simulink model "EVX_Car_Model"  (R2018b)
settings: Solver=VariableStepAuto  StartTime=0.0  StopTime=10.0  RelTol=1e-3
settings Model: Creator=Foster  LastModifiedBy=Foster

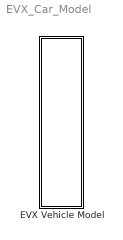
== system EVX_Car_Model ==
  EVX Vehicle Model : Subsystem

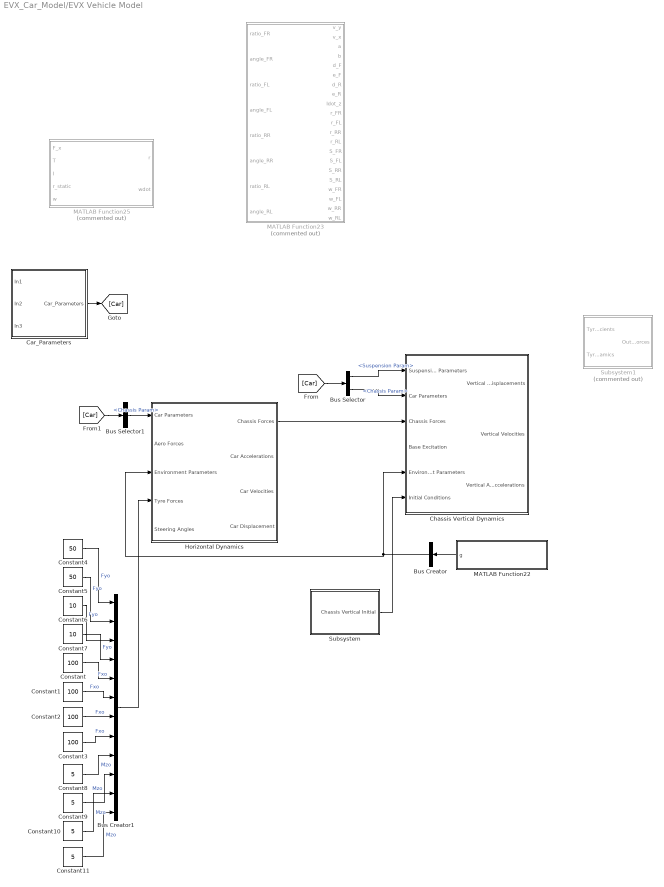
== system EVX_Car_Model/EVX Vehicle Model ==
  Bus Creator : BusCreator  Inputs=1
  Bus Creator1 : BusCreator  Inputs=12
  Bus Selector : BusSelector  OutputSignals=Suspension Param,Chassis Param
  Bus Selector1 : BusSelector  OutputSignals=Chassis Param
  Car_Parameters : Subsystem
  Chassis Vertical Dynamics : Subsystem
  Constant{,1..3} (4 alike) : Constant  Value=100
  Constant{8..11} (4 alike) : Constant  Value=5
  Constant4 : Constant  Value=50
  Constant5 : Constant  Value=50
  Constant6 : Constant  Value=10
  Constant7 : Constant  Value=10
  Horizontal Dynamics : Subsystem
  MATLAB Function22 : MATLAB Function  TreatAsAtomicUnit=on
  MATLAB Function23 : MATLAB Function  Commented=on  TreatAsAtomicUnit=on
  MATLAB Function25 : MATLAB Function  Commented=on  TreatAsAtomicUnit=on
  Subsystem : Subsystem
  Subsystem1 : Subsystem  Commented=on
  wires:
  Subsystem/1(Chassis Vertical Initial) -> Chassis Vertical Dynamics/6(Initial Conditions)
  Constant7/1 -> Bus Creator1/4  "Fyo"
  Constant6/1 -> Bus Creator1/3  "Fyo"
  Constant11/1 -> Bus Creator1/12  "Mzo"
  Bus Creator1/1 -> Horizontal Dynamics/4(Tyre Forces)
  MATLAB Function22/1(g) -> Bus Creator/1
  Constant9/1 -> Bus Creator1/10  "Mzo"
  Constant4/1 -> Bus Creator1/1  "Fyo"
  Bus Selector/1 -> Chassis Vertical Dynamics/1(Suspension Parameters)  "<Suspension Param>"
  Constant3/1 -> Bus Creator1/8  "Fxo"
  Bus Selector1/1 -> Horizontal Dynamics/1(Car Parameters)  "<Chassis Param>"
  [Car] -> Bus Selector/1
  Constant10/1 -> Bus Creator1/11  "Mzo"
  Bus Selector/2 -> Chassis Vertical Dynamics/2(Car Parameters)  "<Chassis Param>"
  Car_Parameters/1(Car_Parameters) -> [Car]
  Horizontal Dynamics/1(Chassis Forces) -> Chassis Vertical Dynamics/3(Chassis Forces)
  [Car] -> Bus Selector1/1
  Constant1/1 -> Bus Creator1/6  "Fxo"
  Constant2/1 -> Bus Creator1/7  "Fxo"
  Bus Creator/1 -> Chassis Vertical Dynamics/5(Environment Parameters), Horizontal Dynamics/3(Environment Parameters)
  Constant/1 -> Bus Creator1/5  "Fxo"
  Constant5/1 -> Bus Creator1/2  "Fyo"
  Constant8/1 -> Bus Creator1/9  "Mzo"

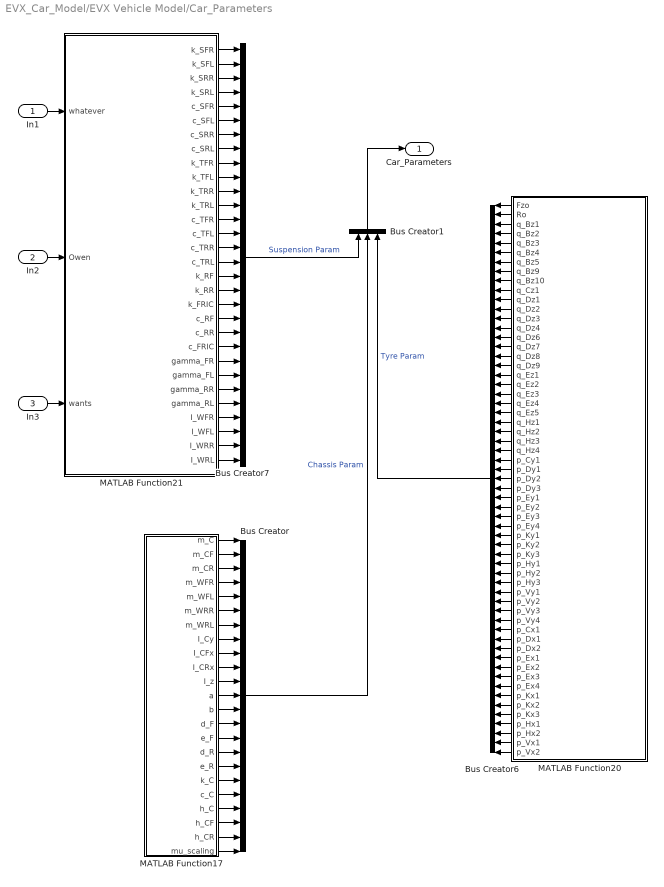
== system EVX_Car_Model/EVX Vehicle Model/Car_Parameters ==
  In1 : Inport
  In2 : Inport  Port=2
  In3 : Inport  Port=3
  Bus Creator : BusCreator  Inputs=23
  Bus Creator1 : BusCreator  Inputs=3
  Bus Creator6 : BusCreator  Inputs=59
  Bus Creator7 : BusCreator  Inputs=30
  MATLAB Function17 : MATLAB Function  TreatAsAtomicUnit=on
  MATLAB Function20 : MATLAB Function  TreatAsAtomicUnit=on
  MATLAB Function21 : MATLAB Function  TreatAsAtomicUnit=on
  Car_Parameters : Outport
  wires:
  In1/1 -> MATLAB Function21/1(whatever)
  In2/1 -> MATLAB Function21/2(Owen)
  In3/1 -> MATLAB Function21/3(wants)
  MATLAB Function21/1(k_SFR) -> Bus Creator7/1
  MATLAB Function21/2(k_SFL) -> Bus Creator7/2
  MATLAB Function21/3(k_SRR) -> Bus Creator7/3
  MATLAB Function21/4(k_SRL) -> Bus Creator7/4
  MATLAB Function21/5(c_SFR) -> Bus Creator7/5
  MATLAB Function21/6(c_SFL) -> Bus Creator7/6
  MATLAB Function21/7(c_SRR) -> Bus Creator7/7
  MATLAB Function21/8(c_SRL) -> Bus Creator7/8
  MATLAB Function21/9(k_TFR) -> Bus Creator7/9
  MATLAB Function21/10(k_TFL) -> Bus Creator7/10
  MATLAB Function21/11(k_TRR) -> Bus Creator7/11
  MATLAB Function21/12(k_TRL) -> Bus Creator7/12
  MATLAB Function21/13(c_TFR) -> Bus Creator7/13
  MATLAB Function21/14(c_TFL) -> Bus Creator7/14
  MATLAB Function21/15(c_TRR) -> Bus Creator7/15
  MATLAB Function21/16(c_TRL) -> Bus Creator7/16
  MATLAB Function21/17(k_RF) -> Bus Creator7/17
  MATLAB Function21/18(k_RR) -> Bus Creator7/18
  MATLAB Function21/19(k_FRIC) -> Bus Creator7/19
  MATLAB Function21/20(c_RF) -> Bus Creator7/20
  MATLAB Function21/21(c_RR) -> Bus Creator7/21
  MATLAB Function21/22(c_FRIC) -> Bus Creator7/22
  MATLAB Function21/23(gamma_FR) -> Bus Creator7/23
  MATLAB Function21/24(gamma_FL) -> Bus Creator7/24
  MATLAB Function21/25(gamma_RR) -> Bus Creator7/25
  MATLAB Function21/26(gamma_RL) -> Bus Creator7/26
  MATLAB Function21/27(I_WFR) -> Bus Creator7/27
  MATLAB Function21/28(I_WFL) -> Bus Creator7/28
  MATLAB Function21/29(I_WRR) -> Bus Creator7/29
  MATLAB Function21/30(I_WRL) -> Bus Creator7/30
  MATLAB Function17/1(m_C) -> Bus Creator/1
  MATLAB Function17/2(m_CF) -> Bus Creator/2
  MATLAB Function17/3(m_CR) -> Bus Creator/3
  MATLAB Function17/4(m_WFR) -> Bus Creator/4
  MATLAB Function17/5(m_WFL) -> Bus Creator/5
  MATLAB Function17/6(m_WRR) -> Bus Creator/6
  MATLAB Function17/7(m_WRL) -> Bus Creator/7
  MATLAB Function17/8(I_Cy) -> Bus Creator/8
  MATLAB Function17/9(I_CFx) -> Bus Creator/9
  MATLAB Function17/10(I_CRx) -> Bus Creator/10
  MATLAB Function17/11(I_z) -> Bus Creator/11
  MATLAB Function17/12(a) -> Bus Creator/12
  MATLAB Function17/13(b) -> Bus Creator/13
  MATLAB Function17/14(d_F) -> Bus Creator/14
  MATLAB Function17/15(e_F) -> Bus Creator/15
  MATLAB Function17/16(d_R) -> Bus Creator/16
  MATLAB Function17/17(e_R) -> Bus Creator/17
  MATLAB Function17/18(k_C) -> Bus Creator/18
  MATLAB Function17/19(c_C) -> Bus Creator/19
  MATLAB Function17/20(h_C) -> Bus Creator/20
  MATLAB Function17/21(h_CF) -> Bus Creator/21
  MATLAB Function17/22(h_CR) -> Bus Creator/22
  MATLAB Function17/23(mu_scaling) -> Bus Creator/23
  MATLAB Function20/1(Fzo) -> Bus Creator6/1
  MATLAB Function20/59(p_Vx2) -> Bus Creator6/59
  MATLAB Function20/58(p_Vx1) -> Bus Creator6/58
  MATLAB Function20/57(p_Hx2) -> Bus Creator6/57
  MATLAB Function20/56(p_Hx1) -> Bus Creator6/56
  MATLAB Function20/55(p_Kx3) -> Bus Creator6/55
  MATLAB Function20/54(p_Kx2) -> Bus Creator6/54
  MATLAB Function20/53(p_Kx1) -> Bus Creator6/53
  MATLAB Function20/52(p_Ex4) -> Bus Creator6/52
  MATLAB Function20/51(p_Ex3) -> Bus Creator6/51
  MATLAB Function20/50(p_Ex2) -> Bus Creator6/50
  MATLAB Function20/49(p_Ex1) -> Bus Creator6/49
  MATLAB Function20/48(p_Dx2) -> Bus Creator6/48
  MATLAB Function20/47(p_Dx1) -> Bus Creator6/47
  MATLAB Function20/46(p_Cx1) -> Bus Creator6/46
  MATLAB Function20/45(p_Vy4) -> Bus Creator6/45
  MATLAB Function20/44(p_Vy3) -> Bus Creator6/44
  MATLAB Function20/43(p_Vy2) -> Bus Creator6/43
  MATLAB Function20/42(p_Vy1) -> Bus Creator6/42
  MATLAB Function20/41(p_Hy3) -> Bus Creator6/41
  MATLAB Function20/39(p_Hy1) -> Bus Creator6/39
  MATLAB Function20/40(p_Hy2) -> Bus Creator6/40
  MATLAB Function20/38(p_Ky3) -> Bus Creator6/38
  MATLAB Function20/37(p_Ky2) -> Bus Creator6/37
  MATLAB Function20/36(p_Ky1) -> Bus Creator6/36
  MATLAB Function20/35(p_Ey4) -> Bus Creator6/35
  MATLAB Function20/34(p_Ey3) -> Bus Creator6/34
  MATLAB Function20/33(p_Ey2) -> Bus Creator6/33
  MATLAB Function20/32(p_Ey1) -> Bus Creator6/32
  MATLAB Function20/31(p_Dy3) -> Bus Creator6/31
  MATLAB Function20/2(Ro) -> Bus Creator6/2
  MATLAB Function20/3(q_Bz1) -> Bus Creator6/3
  MATLAB Function20/4(q_Bz2) -> Bus Creator6/4
  MATLAB Function20/5(q_Bz3) -> Bus Creator6/5
  MATLAB Function20/6(q_Bz4) -> Bus Creator6/6
  MATLAB Function20/7(q_Bz5) -> Bus Creator6/7
  MATLAB Function20/8(q_Bz9) -> Bus Creator6/8
  MATLAB Function20/9(q_Bz10) -> Bus Creator6/9
  MATLAB Function20/10(q_Cz1) -> Bus Creator6/10
  MATLAB Function20/11(q_Dz1) -> Bus Creator6/11
  MATLAB Function20/12(q_Dz2) -> Bus Creator6/12
  MATLAB Function20/13(q_Dz3) -> Bus Creator6/13
  MATLAB Function20/14(q_Dz4) -> Bus Creator6/14
  MATLAB Function20/15(q_Dz6) -> Bus Creator6/15
  MATLAB Function20/16(q_Dz7) -> Bus Creator6/16
  MATLAB Function20/17(q_Dz8) -> Bus Creator6/17
  MATLAB Function20/18(q_Dz9) -> Bus Creator6/18
  MATLAB Function20/19(q_Ez1) -> Bus Creator6/19
  MATLAB Function20/20(q_Ez2) -> Bus Creator6/20
  MATLAB Function20/21(q_Ez3) -> Bus Creator6/21
  MATLAB Function20/22(q_Ez4) -> Bus Creator6/22
  MATLAB Function20/23(q_Ez5) -> Bus Creator6/23
  MATLAB Function20/24(q_Hz1) -> Bus Creator6/24
  MATLAB Function20/25(q_Hz2) -> Bus Creator6/25
  MATLAB Function20/26(q_Hz3) -> Bus Creator6/26
  MATLAB Function20/27(q_Hz4) -> Bus Creator6/27
  MATLAB Function20/28(p_Cy1) -> Bus Creator6/28
  MATLAB Function20/29(p_Dy1) -> Bus Creator6/29
  MATLAB Function20/30(p_Dy2) -> Bus Creator6/30
  Bus Creator7/1 -> Bus Creator1/1  "Suspension Param"
  Bus Creator/1 -> Bus Creator1/2  "Chassis Param"
  Bus Creator6/1 -> Bus Creator1/3  "Tyre Param"
  Bus Creator1/1 -> Car_Parameters/1

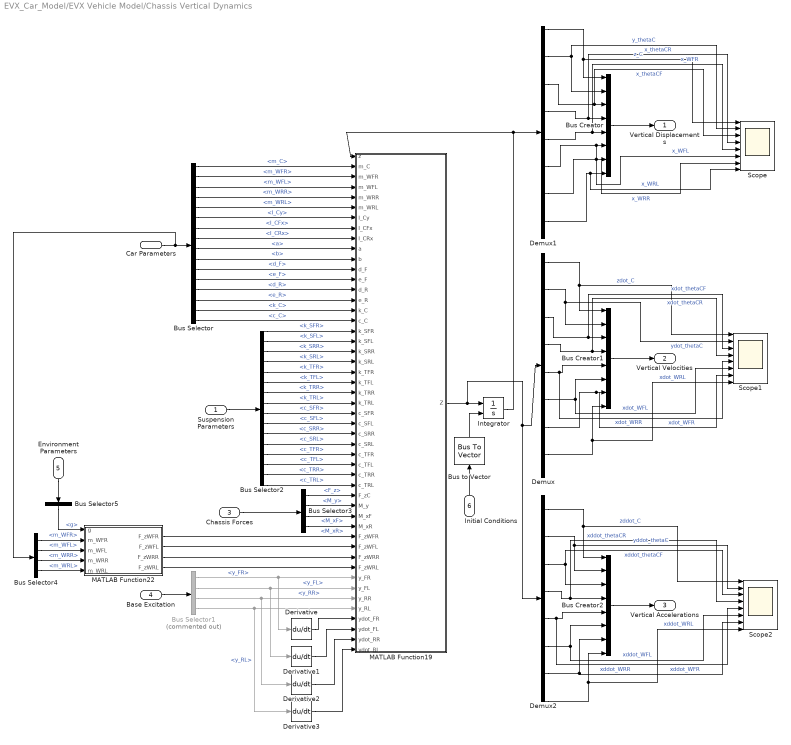
== system EVX_Car_Model/EVX Vehicle Model/Chassis Vertical Dynamics ==
  Suspension Parameters : Inport
  Car Parameters : Inport  Port=2
  Chassis Forces : Inport  Port=3
  Base Excitation : Inport  Port=4
  Environment Parameters : Inport  Port=5
  Initial Conditions : Inport  Port=6
  Bus Creator : BusCreator  Inputs=8
  Bus Creator1 : BusCreator  Inputs=8
  Bus Creator2 : BusCreator  Inputs=8
  Bus Selector : BusSelector  OutputSignals=m_C,m_WFR,m_WFL,m_WRR,m_WRL,I_Cy,I_CFx,I_CRx,a,b,d_F,e_F,d_R,e_R,k_C,c_C
  Bus Selector1 : BusSelector  Commented=on  OutputSignals=y_FR,y_FL,y_RR,y_RL
  Bus Selector2 : BusSelector  OutputSignals=k_SFR,k_SFL,k_SRR,k_SRL,k_TFR,k_TFL,k_TRR,k_TRL,c_SFR,c_SFL,c_SRR,c_SRL,c_TFR,c_TFL,c_TRR,c_TRL
  Bus Selector3 : BusSelector  OutputSignals=F_z,M_y,M_xF,M_xR
  Bus Selector4 : BusSelector  OutputSignals=m_WFR,m_WFL,m_WRR,m_WRL
  Bus Selector5 : BusSelector  OutputSignals=g
  Bus to Vector : BusToVector
  Demux : Demux  Outputs=16
  Demux1 : Demux  Outputs=16
  Demux2 : Demux  Outputs=16
  Derivative{,1..3} (4 alike) : Derivative
  Integrator : Integrator  InitialConditionSource=external
  MATLAB Function19 : MATLAB Function  TreatAsAtomicUnit=on
  MATLAB Function22 : MATLAB Function  TreatAsAtomicUnit=on
  Scope : Scope  NumInputPorts=8
  Scope1 : Scope  NumInputPorts=8
  Scope2 : Scope  NumInputPorts=8
  Vertical Displacements : Outport
  Vertical Velocities : Outport  Port=2
  Vertical Accelerations : Outport  Port=3
  wires:
  Car Parameters/1 -> Bus Selector4/1, Bus Selector/1
  Bus Selector/1 -> MATLAB Function19/2(m_C)  "<m_C>"
  Bus Selector/2 -> MATLAB Function19/3(m_WFR)  "<m_WFR>"
  Bus Selector/3 -> MATLAB Function19/4(m_WFL)  "<m_WFL>"
  Bus Selector/4 -> MATLAB Function19/5(m_WRR)  "<m_WRR>"
  Bus Selector/5 -> MATLAB Function19/6(m_WRL)  "<m_WRL>"
  Bus Selector/6 -> MATLAB Function19/7(I_Cy)  "<I_Cy>"
  Bus Selector/7 -> MATLAB Function19/8(I_CFx)  "<I_CFx>"
  Bus Selector/8 -> MATLAB Function19/9(I_CRx)  "<I_CRx>"
  Bus Selector/9 -> MATLAB Function19/10(a)  "<a>"
  MATLAB Function19/1(Z) -> Demux2/1, Demux/1, Integrator/1
  Demux1/1 -> Bus Creator/1, Scope/1  "z_C"
  Demux1/3 -> Bus Creator/2, Scope/2  "y_thetaC"
  Demux1/5 -> Scope/3, Bus Creator/3  "x_thetaCF"
  Demux1/7 -> Scope/4, Bus Creator/4  "x_thetaCR"
  Demux1/9 -> Scope/5, Bus Creator/5  "x_WFR"
  Demux1/11 -> Scope/6, Bus Creator/6  "x_WFL"
  Demux1/13 -> Scope/7, Bus Creator/7  "x_WRR"
  Demux1/15 -> Scope/8, Bus Creator/8  "x_WRL"
  Bus Creator/1 -> Vertical Displacements/1
  Bus Creator1/1 -> Vertical Velocities/1
  Bus Creator2/1 -> Vertical Accelerations/1
  Demux/1 -> Scope1/1, Bus Creator1/1  "zdot_C"
  Demux/3 -> Scope1/2, Bus Creator1/2  "ydot_thetaC"
  Demux/5 -> Scope1/3, Bus Creator1/3  "xdot_thetaCF"
  Demux/7 -> Scope1/4, Bus Creator1/4  "xdot_thetaCR"
  Demux/9 -> Scope1/5, Bus Creator1/5  "xdot_WFR"
  Demux/11 -> Bus Creator1/6, Scope1/6  "xdot_WFL"
  Demux/13 -> Scope1/7, Bus Creator1/7  "xdot_WRR"
  Demux/15 -> Scope1/8, Bus Creator1/8  "xdot_WRL"
  Demux2/2 -> Scope2/1, Bus Creator2/1  "zddot_C"
  Demux2/4 -> Bus Creator2/2, Scope2/2  "yddot_thetaC"
  Demux2/6 -> Bus Creator2/3, Scope2/3  "xddot_thetaCF"
  Demux2/8 -> Scope2/4, Bus Creator2/4  "xddot_thetaCR"
  Demux2/10 -> Scope2/5, Bus Creator2/5  "xddot_WFR"
  Demux2/12 -> Bus Creator2/6, Scope2/6  "xddot_WFL"
  Demux2/14 -> Bus Creator2/7, Scope2/7  "xddot_WRR"
  Demux2/16 -> Scope2/8, Bus Creator2/8  "xddot_WRL"
  Base Excitation/1 -> Bus Selector1/1
  Bus Selector1/1 -> Derivative/1, MATLAB Function19/42(y_FR)  "<y_FR>"
  Bus Selector1/2 -> Derivative1/1, MATLAB Function19/43(y_FL)  "<y_FL>"
  Bus Selector1/3 -> Derivative2/1, MATLAB Function19/44(y_RR)  "<y_RR>"
  Bus Selector1/4 -> Derivative3/1, MATLAB Function19/45(y_RL)  "<y_RL>"
  Derivative/1 -> MATLAB Function19/46(ydot_FR)
  Derivative1/1 -> MATLAB Function19/47(ydot_FL)
  Derivative2/1 -> MATLAB Function19/48(ydot_RR)
  Derivative3/1 -> MATLAB Function19/49(ydot_RL)
  Suspension Parameters/1 -> Bus Selector2/1
  Bus Selector2/1 -> MATLAB Function19/18(k_SFR)  "<k_SFR>"
  Bus Selector2/2 -> MATLAB Function19/19(k_SFL)  "<k_SFL>"
  Bus Selector2/3 -> MATLAB Function19/20(k_SRR)  "<k_SRR>"
  Bus Selector2/4 -> MATLAB Function19/21(k_SRL)  "<k_SRL>"
  Bus Selector2/9 -> MATLAB Function19/26(c_SFR)  "<c_SFR>"
  Bus Selector2/10 -> MATLAB Function19/27(c_SFL)  "<c_SFL>"
  Bus Selector2/11 -> MATLAB Function19/28(c_SRR)  "<c_SRR>"
  Bus Selector2/12 -> MATLAB Function19/29(c_SRL)  "<c_SRL>"
  Bus Selector2/5 -> MATLAB Function19/22(k_TFR)  "<k_TFR>"
  Bus Selector2/6 -> MATLAB Function19/23(k_TFL)  "<k_TFL>"
  Bus Selector2/7 -> MATLAB Function19/24(k_TRR)  "<k_TRR>"
  Bus Selector2/8 -> MATLAB Function19/25(k_TRL)  "<k_TRL>"
  Bus Selector2/13 -> MATLAB Function19/30(c_TFR)  "<c_TFR>"
  Bus Selector2/14 -> MATLAB Function19/31(c_TFL)  "<c_TFL>"
  Bus Selector2/15 -> MATLAB Function19/32(c_TRR)  "<c_TRR>"
  Bus Selector2/16 -> MATLAB Function19/33(c_TRL)  "<c_TRL>"
  Chassis Forces/1 -> Bus Selector3/1
  Bus Selector3/1 -> MATLAB Function19/34(F_zC)  "<F_z>"
  Bus Selector3/2 -> MATLAB Function19/35(M_y)  "<M_y>"
  Bus Selector3/3 -> MATLAB Function19/36(M_xF)  "<M_xF>"
  Bus Selector3/4 -> MATLAB Function19/37(M_xR)  "<M_xR>"
  Bus Selector4/1 -> MATLAB Function22/2(m_WFR)  "<m_WFR>"
  Bus Selector4/2 -> MATLAB Function22/3(m_WFL)  "<m_WFL>"
  Bus Selector4/3 -> MATLAB Function22/4(m_WRR)  "<m_WRR>"
  Bus Selector4/4 -> MATLAB Function22/5(m_WRL)  "<m_WRL>"
  Environment Parameters/1 -> Bus Selector5/1
  MATLAB Function22/1(F_zWFR) -> MATLAB Function19/38(F_zWFR)
  MATLAB Function22/2(F_zWFL) -> MATLAB Function19/39(F_zWFL)
  MATLAB Function22/3(F_zWRR) -> MATLAB Function19/40(F_zWRR)
  MATLAB Function22/4(F_zWRL) -> MATLAB Function19/41(F_zWRL)
  Bus Selector5/1 -> MATLAB Function22/1(g)  "<g>"
  Bus Selector/10 -> MATLAB Function19/11(b)  "<b>"
  Bus Selector/11 -> MATLAB Function19/12(d_F)  "<d_F>"
  Bus Selector/12 -> MATLAB Function19/13(e_F)  "<e_F>"
  Bus Selector/13 -> MATLAB Function19/14(d_R)  "<d_R>"
  Bus Selector/14 -> MATLAB Function19/15(e_R)  "<e_R>"
  Bus Selector/15 -> MATLAB Function19/16(k_C)  "<k_C>"
  Bus Selector/16 -> MATLAB Function19/17(c_C)  "<c_C>"
  Integrator/1 -> MATLAB Function19/1(z), Demux1/1
  Initial Conditions/1 -> Bus to Vector/1
  Bus to Vector/1 -> Integrator/2

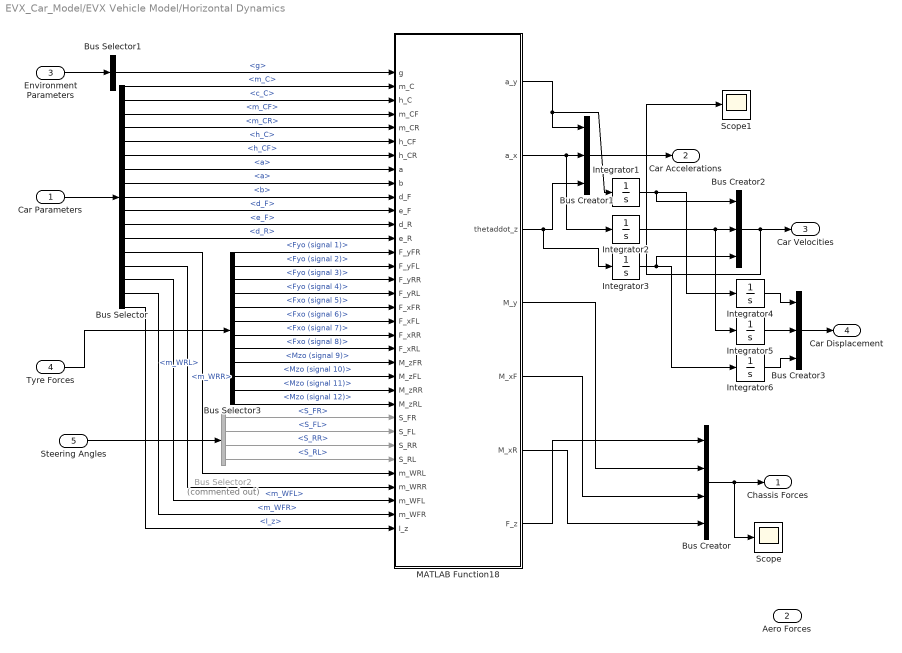
== system EVX_Car_Model/EVX Vehicle Model/Horizontal Dynamics ==
  Car Parameters : Inport
  Aero Forces : Inport  Port=2
  Environment Parameters : Inport  Port=3
  Tyre Forces : Inport  Port=4
  Steering Angles : Inport  Port=5
  Bus Creator : BusCreator  Inputs=4
  Bus Creator1 : BusCreator  Inputs=3
  Bus Creator2 : BusCreator  Inputs=3
  Bus Creator3 : BusCreator  Inputs=3
  Bus Selector : BusSelector  OutputSignals=m_C,c_C,m_CF,m_CR,h_C,h_CF,a,a,b,d_F,e_F,d_R,m_WRL,m_WRR,m_WFL,m_WFR,I_z
  Bus Selector1 : BusSelector  OutputSignals=g
  Bus Selector2 : BusSelector  Commented=on  OutputSignals=S_FR,S_FL,S_RR,S_RL
  Bus Selector3 : BusSelector  OutputSignals=Fyo (signal 1),Fyo (signal 2),Fyo (signal 3),Fyo (signal 4),Fxo (signal 5),Fxo (signal 6),Fxo (signal 7),Fxo (signal 8),Mzo (signal 9),Mzo (signal 10),Mzo (signal 11),Mzo (signal 12)
  Integrator{1..6} (6 alike) : Integrator
  MATLAB Function18 : MATLAB Function  TreatAsAtomicUnit=on
  Scope : Scope
  Scope1 : Scope
  Chassis Forces : Outport
  Car Accelerations : Outport  Port=2
  Car Velocities : Outport  Port=3
  Car Displacement : Outport  Port=4
  wires:
  MATLAB Function18/7(F_z) -> Bus Creator/1
  MATLAB Function18/4(M_y) -> Bus Creator/2
  MATLAB Function18/5(M_xF) -> Bus Creator/3
  MATLAB Function18/6(M_xR) -> Bus Creator/4
  Bus Creator/1 -> Scope/1, Chassis Forces/1
  Car Parameters/1 -> Bus Selector/1
  Bus Selector/1 -> MATLAB Function18/2(m_C)  "<m_C>"
  Bus Selector/2 -> MATLAB Function18/3(h_C)  "<c_C>"
  Bus Selector/3 -> MATLAB Function18/4(m_CF)  "<m_CF>"
  Bus Selector/4 -> MATLAB Function18/5(m_CR)  "<m_CR>"
  Bus Selector/5 -> MATLAB Function18/6(h_CF)  "<h_C>"
  Bus Selector/6 -> MATLAB Function18/7(h_CR)  "<h_CF>"
  Bus Selector/7 -> MATLAB Function18/8(a)  "<a>"
  Bus Selector/8 -> MATLAB Function18/9(b)  "<a>"
  Bus Selector/9 -> MATLAB Function18/10(d_F)  "<b>"
  Bus Selector/10 -> MATLAB Function18/11(e_F)  "<d_F>"
  Bus Selector/11 -> MATLAB Function18/12(d_R)  "<e_F>"
  Bus Selector/12 -> MATLAB Function18/13(e_R)  "<d_R>"
  Bus Selector/16 -> MATLAB Function18/33(m_WFR)  "<m_WFR>"
  Bus Selector/15 -> MATLAB Function18/32(m_WFL)  "<m_WFL>"
  Bus Selector/14 -> MATLAB Function18/31(m_WRR)  "<m_WRR>"
  Bus Selector/13 -> MATLAB Function18/30(m_WRL)  "<m_WRL>"
  Bus Selector/17 -> MATLAB Function18/34(I_z)  "<I_z>"
  Bus Creator1/1 -> Car Accelerations/1
  MATLAB Function18/2(a_x) -> Integrator2/1, Bus Creator1/2
  MATLAB Function18/1(a_y) -> Integrator1/1, Bus Creator1/1
  MATLAB Function18/3(thetaddot_z) -> Integrator3/1, Bus Creator1/3
  Environment Parameters/1 -> Bus Selector1/1
  Bus Selector1/1 -> MATLAB Function18/1(g)  "<g>"
  Integrator2/1 -> Integrator5/1, Bus Creator2/2
  Integrator1/1 -> Integrator4/1, Bus Creator2/1
  Integrator3/1 -> Integrator6/1, Bus Creator2/3
  Bus Creator2/1 -> Scope1/1, Car Velocities/1
  Integrator4/1 -> Bus Creator3/1
  Integrator6/1 -> Bus Creator3/3
  Integrator5/1 -> Bus Creator3/2
  Bus Creator3/1 -> Car Displacement/1
  Steering Angles/1 -> Bus Selector2/1
  Tyre Forces/1 -> Bus Selector3/1
  Bus Selector2/1 -> MATLAB Function18/26(S_FR)  "<S_FR>"
  Bus Selector2/2 -> MATLAB Function18/27(S_FL)  "<S_FL>"
  Bus Selector2/3 -> MATLAB Function18/28(S_RR)  "<S_RR>"
  Bus Selector2/4 -> MATLAB Function18/29(S_RL)  "<S_RL>"
  Bus Selector3/1 -> MATLAB Function18/14(F_yFR)  "<Fyo (signal 1)>"
  Bus Selector3/2 -> MATLAB Function18/15(F_yFL)  "<Fyo (signal 2)>"
  Bus Selector3/3 -> MATLAB Function18/16(F_yRR)  "<Fyo (signal 3)>"
  Bus Selector3/4 -> MATLAB Function18/17(F_yRL)  "<Fyo (signal 4)>"
  Bus Selector3/5 -> MATLAB Function18/18(F_xFR)  "<Fxo (signal 5)>"
  Bus Selector3/6 -> MATLAB Function18/19(F_xFL)  "<Fxo (signal 6)>"
  Bus Selector3/7 -> MATLAB Function18/20(F_xRR)  "<Fxo (signal 7)>"
  Bus Selector3/8 -> MATLAB Function18/21(F_xRL)  "<Fxo (signal 8)>"
  Bus Selector3/9 -> MATLAB Function18/22(M_zFR)  "<Mzo (signal 9)>"
  Bus Selector3/10 -> MATLAB Function18/23(M_zFL)  "<Mzo (signal 10)>"
  Bus Selector3/11 -> MATLAB Function18/24(M_zRR)  "<Mzo (signal 11)>"
  Bus Selector3/12 -> MATLAB Function18/25(M_zRL)  "<Mzo (signal 12)>"

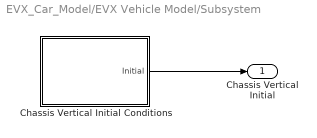
== system EVX_Car_Model/EVX Vehicle Model/Subsystem ==
  Chassis Vertical Initial Conditions : MATLAB Function  TreatAsAtomicUnit=on
  Chassis Vertical Initial : Outport
  wires:
  Chassis Vertical Initial Conditions/1(Initial) -> Chassis Vertical Initial/1

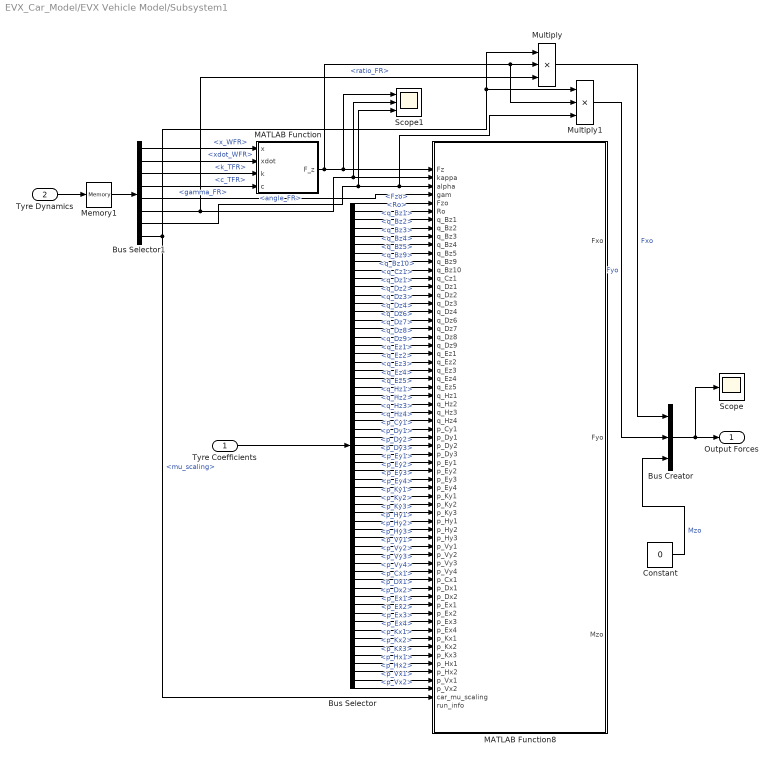
== system EVX_Car_Model/EVX Vehicle Model/Subsystem1 ==
  Tyre Coefficients : Inport
  Tyre Dynamics : Inport  Port=2
  Bus Creator : BusCreator  Inputs=3
  Bus Selector : BusSelector  OutputSignals=Fzo,Ro,q_Bz1,q_Bz2,q_Bz3,q_Bz4,q_Bz5,q_Bz9,q_Bz10,q_Cz1,q_Dz1,q_Dz2,q_Dz3,q_Dz4,q_Dz6,q_Dz7,q_Dz8,q_Dz9,q_Ez1,q_Ez2,q_Ez3,q_Ez4,q_Ez5,q_Hz1,q_Hz2,q_Hz3,q_Hz4,p_Cy1,p_Dy1,p_Dy2,p_Dy3,p_Ey1,p_Ey2,p_Ey3,p_Ey4,p_Ky1,p_Ky2,p_Ky3,p_Hy1,p_Hy2,p_Hy3,p_Vy1,p_Vy2,p_Vy3,p_Vy4,p_Cx1,p_Dx1,p_Dx2,p_Ex1,p_Ex2,p_Ex3,p_Ex4,p_Kx1,p_Kx2,p_Kx3,p_Hx1,p_Hx2,p_Vx1,p_Vx2
  Bus Selector1 : BusSelector  OutputSignals=x_WFR,xdot_WFR,signal3.k_TFR,signal3.c_TFR,signal3.gamma_FR,signal4.ratio_FR,signal4.angle_FR,mu_scaling
  Constant : Constant  Value=0
  MATLAB Function : MATLAB Function  TreatAsAtomicUnit=on
  MATLAB Function8 : MATLAB Function  TreatAsAtomicUnit=on
  Memory1 : Memory
  Multiply : Product  Inputs=3
  Multiply1 : Product  Inputs=3
  Scope : Scope
  Scope1 : Scope  NumInputPorts=3
  Output Forces : Outport
  wires:
  Bus Creator/1 -> Scope/1, Output Forces/1
  Tyre Coefficients/1 -> Bus Selector/1
  Bus Selector/1 -> MATLAB Function8/5(Fzo)  "<Fzo>"
  Bus Selector/2 -> MATLAB Function8/6(Ro)  "<Ro>"
  Tyre Dynamics/1 -> Memory1/1
  Bus Selector1/1 -> MATLAB Function/1(x)  "<x_WFR>"
  Bus Selector1/2 -> MATLAB Function/2(xdot)  "<xdot_WFR>"
  MATLAB Function/1(F_z) -> Multiply1/2, Multiply/2, Scope1/1, MATLAB Function8/1(Fz)
  Bus Selector1/3 -> MATLAB Function/3(k)  "<k_TFR>"
  Bus Selector1/4 -> MATLAB Function/4(c)  "<c_TFR>"
  Bus Selector1/5 -> MATLAB Function8/4(gam)  "<gamma_FR>"
  Bus Selector/3 -> MATLAB Function8/7(q_Bz1)  "<q_Bz1>"
  Bus Selector/4 -> MATLAB Function8/8(q_Bz2)  "<q_Bz2>"
  Bus Selector/5 -> MATLAB Function8/9(q_Bz3)  "<q_Bz3>"
  Bus Selector/6 -> MATLAB Function8/10(q_Bz4)  "<q_Bz4>"
  Bus Selector/7 -> MATLAB Function8/11(q_Bz5)  "<q_Bz5>"
  Bus Selector/8 -> MATLAB Function8/12(q_Bz9)  "<q_Bz9>"
  Bus Selector/9 -> MATLAB Function8/13(q_Bz10)  "<q_Bz10>"
  Bus Selector/10 -> MATLAB Function8/14(q_Cz1)  "<q_Cz1>"
  Bus Selector/11 -> MATLAB Function8/15(q_Dz1)  "<q_Dz1>"
  Bus Selector/12 -> MATLAB Function8/16(q_Dz2)  "<q_Dz2>"
  Bus Selector/13 -> MATLAB Function8/17(q_Dz3)  "<q_Dz3>"
  Bus Selector/14 -> MATLAB Function8/18(q_Dz4)  "<q_Dz4>"
  Bus Selector/15 -> MATLAB Function8/19(q_Dz6)  "<q_Dz6>"
  Bus Selector/16 -> MATLAB Function8/20(q_Dz7)  "<q_Dz7>"
  Bus Selector/17 -> MATLAB Function8/21(q_Dz8)  "<q_Dz8>"
  Bus Selector/18 -> MATLAB Function8/22(q_Dz9)  "<q_Dz9>"
  Bus Selector/19 -> MATLAB Function8/23(q_Ez1)  "<q_Ez1>"
  Bus Selector/20 -> MATLAB Function8/24(q_Ez2)  "<q_Ez2>"
  Bus Selector/21 -> MATLAB Function8/25(q_Ez3)  "<q_Ez3>"
  Bus Selector/22 -> MATLAB Function8/26(q_Ez4)  "<q_Ez4>"
  Bus Selector/23 -> MATLAB Function8/27(q_Ez5)  "<q_Ez5>"
  Bus Selector/24 -> MATLAB Function8/28(q_Hz1)  "<q_Hz1>"
  Bus Selector/25 -> MATLAB Function8/29(q_Hz2)  "<q_Hz2>"
  Bus Selector/26 -> MATLAB Function8/30(q_Hz3)  "<q_Hz3>"
  Bus Selector/27 -> MATLAB Function8/31(q_Hz4)  "<q_Hz4>"
  Bus Selector/28 -> MATLAB Function8/32(p_Cy1)  "<p_Cy1>"
  Bus Selector/29 -> MATLAB Function8/33(p_Dy1)  "<p_Dy1>"
  Bus Selector/30 -> MATLAB Function8/34(p_Dy2)  "<p_Dy2>"
  Bus Selector/31 -> MATLAB Function8/35(p_Dy3)  "<p_Dy3>"
  Bus Selector/32 -> MATLAB Function8/36(p_Ey1)  "<p_Ey1>"
  Bus Selector/33 -> MATLAB Function8/37(p_Ey2)  "<p_Ey2>"
  Bus Selector/34 -> MATLAB Function8/38(p_Ey3)  "<p_Ey3>"
  Bus Selector/35 -> MATLAB Function8/39(p_Ey4)  "<p_Ey4>"
  Bus Selector/36 -> MATLAB Function8/40(p_Ky1)  "<p_Ky1>"
  Bus Selector/37 -> MATLAB Function8/41(p_Ky2)  "<p_Ky2>"
  Bus Selector/38 -> MATLAB Function8/42(p_Ky3)  "<p_Ky3>"
  Bus Selector/39 -> MATLAB Function8/43(p_Hy1)  "<p_Hy1>"
  Bus Selector/40 -> MATLAB Function8/44(p_Hy2)  "<p_Hy2>"
  Bus Selector/41 -> MATLAB Function8/45(p_Hy3)  "<p_Hy3>"
  Bus Selector/42 -> MATLAB Function8/46(p_Vy1)  "<p_Vy1>"
  Bus Selector/43 -> MATLAB Function8/47(p_Vy2)  "<p_Vy2>"
  Bus Selector/44 -> MATLAB Function8/48(p_Vy3)  "<p_Vy3>"
  Bus Selector/45 -> MATLAB Function8/49(p_Vy4)  "<p_Vy4>"
  Bus Selector/46 -> MATLAB Function8/50(p_Cx1)  "<p_Cx1>"
  Bus Selector/47 -> MATLAB Function8/51(p_Dx1)  "<p_Dx1>"
  Bus Selector/48 -> MATLAB Function8/52(p_Dx2)  "<p_Dx2>"
  Bus Selector/49 -> MATLAB Function8/53(p_Ex1)  "<p_Ex1>"
  Bus Selector/50 -> MATLAB Function8/54(p_Ex2)  "<p_Ex2>"
  Bus Selector/51 -> MATLAB Function8/55(p_Ex3)  "<p_Ex3>"
  Bus Selector/52 -> MATLAB Function8/56(p_Ex4)  "<p_Ex4>"
  Bus Selector/53 -> MATLAB Function8/57(p_Kx1)  "<p_Kx1>"
  Bus Selector/54 -> MATLAB Function8/58(p_Kx2)  "<p_Kx2>"
  Bus Selector/55 -> MATLAB Function8/59(p_Kx3)  "<p_Kx3>"
  Bus Selector/56 -> MATLAB Function8/60(p_Hx1)  "<p_Hx1>"
  Bus Selector/57 -> MATLAB Function8/61(p_Hx2)  "<p_Hx2>"
  Bus Selector/58 -> MATLAB Function8/62(p_Vx1)  "<p_Vx1>"
  Bus Selector/59 -> MATLAB Function8/63(p_Vx2)  "<p_Vx2>"
  Bus Selector1/8 -> Multiply1/1, Multiply/1, MATLAB Function8/64(car_mu_scaling)  "<mu_scaling>"
  Bus Selector1/6 -> Multiply/3, Scope1/2, MATLAB Function8/2(kappa)  "<ratio_FR>"
  Bus Selector1/7 -> Scope1/3, MATLAB Function8/3(alpha), Multiply1/3  "<angle_FR>"
  Memory1/1 -> Bus Selector1/1
  Multiply/1 -> Bus Creator/1  "Fxo"
  Multiply1/1 -> Bus Creator/2  "Fyo"
  Constant/1 -> Bus Creator/3  "Mzo"

== matlab function EVX_Car_Model/EVX Vehicle Model/Subsystem/Chassis Vertical Initial Conditions ==
  data: Initial output
function Initial = Chassis_Vertical_Initial()
% Initial Conditions
z_c = -0.25;
y_thetaC = 0;
x_thetaCF = 0;
x_thetaCR = 0;
x_WFR = -0.04;
x_WFL = -0.04;
x_WRR = -0.04;
x_WRL = -0.04;
zdot_c = 0;
ydot_thetaC = 0;
xdot_thetaCF = 0;
xdot_thetaCR = 0;
xdot_WFR = 0;
xdot_WFL = 0;
xdot_WRR = 0;
xdot_WRL = 0;

Initial = [z_c, zdot_c,...
    y_thetaC, ydot_thetaC,...
    x_thetaCF, xdot_thetaCF,...
    x_thetaCR, xdot_thetaCR,...
    x_WFR, xdot_WFR,...
    x_WFL, xdot_WFL,...
    x_WRR, xdot_WRR,...
    x_WRL, xdot_WRL];

== matlab function EVX_Car_Model/EVX Vehicle Model/Car_Parameters/MATLAB Function17 ==
  data: m_C output; m_CF output; m_CR output; m_WFR output; m_WFL output; m_WRR output; m_WRL output; I_Cy output; I_CFx output; I_CRx output; I_z output; a output; b output; d_F output; e_F output; d_R output; e_R output; k_C output; c_C output; h_C output; h_CF output; h_CR output; mu_scaling output
function [m_C,m_CF,m_CR,m_WFR,m_WFL,m_WRR,m_WRL,I_Cy,I_CFx,I_CRx,I_z,a,b,d_F,...
    e_F,d_R,e_R,k_C,c_C,h_C,h_CF,h_CR,mu_scaling] = Car_Parameters
%% Car Parameters
% Masses
m_C = 200; %car sprung mass (kg)
m_CF = 100;
m_CR = m_C - m_CF;
m_WFR = 5; %front right wheel mass (kg)
m_WFL = 5; %front left wheel mass (kg)
m_WRR = 5; %rear right wheel mass (kg)
m_WRL = 5; %rear left wheel mass (kg)

% Intertias
I_Cy = 1000; %chassis interia around y (kg m^2)
I_CFx = 500; %chassis front inertia around x (kg m^2)
I_CRx = 500; %chassis rear inertia around x (kg m^2)
I_z = 2000;

% Geometries
a = 0.8; %distance of COG from front axle (m)
b = 0.8; %distance of COG from rear axle (m)
d_F = 0.6; %distance of COG from front left tire (m)
e_F = 0.6; %distance of COG from front right tire (m)
d_R = 0.6; %distance of COG from rear left tire (m)
e_R = 0.6; %distance of COG from rear right tire (m)
h_C = 0.4;
h_CF = 0.4;
h_CR = 0.4;

% Other Stiffnesses
k_C = 2000;

% Other Damping Coefficients
c_C = 1000;

% mu
mu_scaling = 0.5;

== matlab function EVX_Car_Model/EVX Vehicle Model/Chassis Vertical Dynamics/MATLAB Function19 ==
  data: Z output; z input; m_C input; m_WFR input; m_WFL input; m_WRR input; m_WRL input; I_Cy input; I_CFx input; I_CRx input; a input; b input; d_F input; e_F input; d_R input; e_R input; k_C input; c_C input; k_SFR input; k_SFL input; k_SRR input; k_SRL input; k_TFR input; k_TFL input; k_TRR input; k_TRL input; c_SFR input; c_SFL input; c_SRR input; c_SRL input; c_TFR input; c_TFL input; c_TRR input; c_TRL input; F_zC input; M_y input; M_xF input; M_xR input; F_zWFR input; F_zWFL input; F_zWRR input; F_zWRL input; y_FR input; y_FL input; y_RR input; y_RL input; ydot_FR input; ydot_FL input; ydot_RR input; ydot_RL input
function Z = Chassis8(z,m_C,m_WFR,m_WFL,m_WRR,m_WRL,...
    I_Cy,I_CFx,I_CRx,a,b,d_F,e_F,d_R,e_R,k_C,c_C,k_SFR,k_SFL,k_SRR,k_SRL,...
    k_TFR,k_TFL,k_TRR,k_TRL,c_SFR,c_SFL,c_SRR,c_SRL,c_TFR,c_TFL,...
    c_TRR,c_TRL,F_zC,M_y,M_xF,M_xR,F_zWFR,F_zWFL,F_zWRR,F_zWRL,y_FR,...
    y_FL,y_RR,y_RL,ydot_FR,ydot_FL,ydot_RR,ydot_RL)

Z = [z(2);...
    ...
    (1/m_C) * (F_zC...
    + k_SRR * (z(9) - z(1) - b * z(3) + e_R * z(7))...
    + k_SFR * (z(11) - z(1) + a * z(3) + e_F * z(5))...
    + k_SFL * (z(13) - z(1) + a * z(3) - d_F * z(5))...
    + k_SRL * (z(15) - z(1) - b * z(3) - d_R * z(7))...
    + c_SRR * (z(10) - z(2) - b * z(4) + e_R * z(8))...
    + c_SFR * (z(12) - z(2) + a * z(4) + e_F * z(6))...
    + c_SFL * (z(14) - z(2) + a * z(4) - d_F * z(6))...
    + c_SRL * (z(16) - z(2) - b * z(4) - d_R * z(8)));...
    ...
    z(4);...
    ...
    (1/I_Cy) * (M_y...
    + b * k_SRR * (z(9) - z(1) - b * z(3) + e_R * z(7))...
    - a * k_SFR * (z(11) - z(1) + a * z(3) + e_F * z(5))...
    - a * k_SFL * (z(13) - z(1) + a * z(3) - d_F * z(5))...
    + b * k_SRL * (z(15) - z(1) - b * z(3) - d_R * z(7))...
    + b * c_SRR * (z(10) - z(2) - b * z(4) + e_R * z(8))...
    - a * c_SFR * (z(12) - z(2) + a * z(4) + e_F * z(6))...
    - a * c_SFL * (z(14) - z(2) + a * z(4) - d_F * z(6))...
    + b * c_SRL * (z(16) - z(2) - b * z(4) - d_R * z(8)));...
    ...
    z(6);...
    ...
    (1/I_CFx) * (M_xF...
    - e_F * k_SFR * (z(11) - z(1) + a * z(3) + e_F * z(5))...
    + d_F * k_SFL * (z(13) - z(1) + a * z(3) - d_F * z(5))...
    - k_C * (z(5) - z(7))...
    - e_F * c_SFR * (z(12) - z(2) + a * z(4) + e_F * z(6))...
    + d_F * c_SFL * (z(14) - z(2) + a * z(4) - d_F * z(6))...
    - c_C * (z(6) - z(8)));...
    ...
    z(8);...
    ...
    (1/I_CRx) * (M_xR...
    - e_R * k_SRR * (z(9) - z(1) - b * z(3) + e_R * z(7))...
    + d_F * k_SRL * (z(15) - z(1) - b * z(3) - d_R * z(7))...
    + k_C * (z(5) - z(7))...
    - e_R * c_SRR * (z(10) - z(2) - b * z(4) + e_R * z(8))...
    + d_F * c_SRL * (z(16) - z(2) - b * z(4) - d_R * z(8))...
    + c_C * (z(6) - z(8)));...
    ...
    z(10);...
    ...
    (1/m_WRR) * (F_zWRR...
    + k_TRR * (y_RR - z(9))...
    - k_SRR * (z(9) - z(1) - b * z(3) + e_R * z(7))...
    + c_TRR * (ydot_RR - z(10))...
    - c_SRR * (z(10) - z(2) - b * z(4) + e_R * z(8)));...
    ...
    z(12);...
    ...
    (1/m_WFR) * (F_zWFR...
    + k_TFR * (y_FR - z(11))...
    - k_SFR * (z(11) - z(1) + a * z(3) + e_F * z(5))...
    + c_TFR * (ydot_FR - z(12))...
    - c_SFR * (z(12) - z(2) + a * z(4) + e_F * z(6)));...
    ...
    z(14);...
    ...
    (1/m_WFL) * (F_zWFL...
    + k_TFL * (y_FL - z(13))...
    - k_SFL * (z(13) - z(1) + a * z(3) - d_F * z(5))...
    + c_TFL * (ydot_FL - z(14))...
    - c_SFL * (z(14) - z(2) + a * z(4) - d_F * z(6)));...
    ...
    z(16);...
    ...
    (1/m_WRL) * (F_zWRL...
    + k_TRL * (y_RL - z(15))...
    - k_SRL * (z(15) - z(1) - b * z(3) - d_R * z(7))...
    + c_TRL * (ydot_RL - z(16))...
    - c_SRL * (z(16) - z(2) - b * z(4) - d_R * z(8)))...
    ];

end

== matlab function EVX_Car_Model/EVX Vehicle Model/Horizontal Dynamics/MATLAB Function18 ==
  data: g input; a_y output; m_C input; h_C input; m_CF input; m_CR input; h_CF input; h_CR input; a input; b input; d_F input; e_F input; d_R input; e_R input; F_yFR input; F_yFL input; F_yRR input; F_yRL input; F_xFR input; F_xFL input; F_xRR input; F_xRL input; M_zFR input; M_zFL input; M_zRR input; M_zRL input; S_FR input; S_FL input; S_RR input; S_RL input; m_WRL input; m_WRR input; m_WFL input; m_WFR input; a_x output; thetaddot_z output; M_y output; M_xF output; M_xR output; F_z output; I_z input
function [a_y,a_x,thetaddot_z,M_y,M_xF,M_xR,F_z] = Chassis7(g,m_C,h_C,m_CF,m_CR,...
    h_CF,h_CR,a,b,d_F,e_F,d_R,e_R,F_yFR,F_yFL,F_yRR,F_yRL,F_xFR,F_xFL,...
    F_xRR,F_xRL,M_zFR,M_zFL,M_zRR,M_zRL,S_FR,S_FL,S_RR,S_RL,m_WRL,m_WRR,...
    m_WFL,m_WFR,I_z)

F_y = F_yRL * cos(S_RL) + F_yRR * cos(S_RR) + F_yFL * cos(S_FL) + ...
    F_yFR * cos(S_FR)...
     - F_xRL * sin(S_RL) - F_xRR * sin(S_RR) + F_xFL * sin(S_FL) + ...
    F_xFR * sin(S_FR);

F_x = F_xRL * cos(S_RL) + F_xRR * cos(S_RR) + F_xFL * cos(S_FL) + ...
    F_xFR * cos(S_FR)...
     + F_yRL * sin(S_RL) + F_yRR * sin(S_RR) - F_yFL * sin(S_FL) - ...
    F_yFR * sin(S_FR);

F_z = -g * m_C;

M_z = F_xRR * (sin(S_RR) * b + cos(S_RR) * e_R) +...
    F_yRR * (sin(S_RR) * e_R - cos(S_RR) * b) +...
    F_xFR * (cos(S_FR) * e_F + sin(S_FR) * a) +...
    F_yFR * (cos(S_FR) * a - sin(S_FR) * e_F) +...
    F_xFL * (-cos(S_FL) * d_F + sin(S_FL) * a) +...
    F_yFL * (cos(S_FL) * a + sin(S_FL) * d_F) +...
    F_xRL * (-cos(S_RL) * d_R + sin(S_RL) * b) +...
    F_yRL * (-sin(S_RL) * d_R - cos(S_RL) * b) +...
    + M_zFL + M_zRL + M_zRR + M_zFR;

m = m_C + m_WRL + m_WRR + m_WFL + m_WFR;
a_x = F_x / m;
a_y = F_y / m;
thetaddot_z = M_z / I_z;
M_y = -m_C * a_x * h_C;
M_xF = m_CF * a_y * h_CF;
M_xR = m_CR * a_y * h_CR;

== matlab function EVX_Car_Model/EVX Vehicle Model/Car_Parameters/MATLAB Function20 ==
  data: Fzo output; Ro output; q_Bz1 output; q_Bz2 output; q_Bz3 output; q_Bz4 output; q_Bz5 output; q_Bz9 output; q_Bz10 output; q_Cz1 output; q_Dz1 output; q_Dz2 output; q_Dz3 output; q_Dz4 output; q_Dz6 output; q_Dz7 output; q_Dz8 output; q_Dz9 output; q_Ez1 output; q_Ez2 output; q_Ez3 output; q_Ez4 output; q_Ez5 output; q_Hz1 output; q_Hz2 output; q_Hz3 output; q_Hz4 output; p_Cy1 output; p_Dy1 output; p_Dy2 output; p_Dy3 output; p_Ey1 output; p_Ey2 output; p_Ey3 output; p_Ey4 output; p_Ky1 output; p_Ky2 output; p_Ky3 output; p_Hy1 output; p_Hy2 output; p_Hy3 output; p_Vy1 output; p_Vy2 output; p_Vy3 output; p_Vy4 output; p_Cx1 output; p_Dx1 output; p_Dx2 output; p_Ex1 output; p_Ex2 output; p_Ex3 output; p_Ex4 output; p_Kx1 output; p_Kx2 output; p_Kx3 output; p_Hx1 output; p_Hx2 output; p_Vx1 output; p_Vx2 output
function [Fzo,Ro,q_Bz1,q_Bz2,q_Bz3,q_Bz4,q_Bz5,q_Bz9,q_Bz10,q_Cz1,q_Dz1,...
    q_Dz2,q_Dz3,q_Dz4,q_Dz6,q_Dz7,q_Dz8,q_Dz9,q_Ez1,q_Ez2,q_Ez3,q_Ez4,q_Ez5,...
    q_Hz1,q_Hz2,q_Hz3,q_Hz4,p_Cy1,p_Dy1,p_Dy2,p_Dy3,p_Ey1,p_Ey2,p_Ey3,...
    p_Ey4,p_Ky1,p_Ky2,p_Ky3,p_Hy1,p_Hy2,p_Hy3,p_Vy1,p_Vy2,p_Vy3,p_Vy4,...
    p_Cx1,p_Dx1,p_Dx2,p_Ex1,p_Ex2,p_Ex3,p_Ex4,p_Kx1,p_Kx2,p_Kx3,p_Hx1,...
    p_Hx2,p_Vx1,p_Vx2] = Avon_FITO9241
% pacejka model coefficients provided by Stackpole Engineering Services
% for Avon tyre model FITO 9241
% as found in the document 'SES_FSAE_Tiredata_Rev3'
% Specs:
% Size	6.2/20-13
% Pressure 12 psi


Fzo =	1122.74; % N
Ro = 0.25400; % m

% [ALIGNING COEFFICIENTS]
q_Bz1 =	6.11547;
q_Bz2 =	-1.96461;
q_Bz3 =	1.02155;
q_Bz4 =	5.41323;
q_Bz5 =	-7.58049;
q_Bz9 =	0;
q_Bz10 = 0;
q_Cz1 =	1.25000;
q_Dz1 =	0.15275;
q_Dz2 =	-0.00637;
q_Dz3 =	-0.21282;
q_Dz4 =	0.02719;
q_Dz6 =	-0.00145;
q_Dz7 =	0.01039;
q_Dz8 =	-1.03566;
q_Dz9 =	0.24508;
q_Ez1 =	-4.00001;
q_Ez2 =	0;
q_Ez3 =	0.00003;
q_Ez4 =	0.29616;
q_Ez5 =	2.43287;
q_Hz1 =	-0.00124;
q_Hz2 =	-0.00769;
q_Hz3 =	0.49190;
q_Hz4 =	0.13660;

%  [LATERAL COEFFICIENTS]
p_Cy1 =	0.95232;
p_Dy1 =	2.65462;
p_Dy2 =	0.05198;
p_Dy3 =	-13.51679;
p_Ey1 =	0.29170;
p_Ey2 =	0.30617;
p_Ey3 =	-0.53331;
p_Ey4 =	1.52410;
p_Ky1 =	-27.31900;
p_Ky2 =	-1.06469;
p_Ky3 =	2.27460;
p_Hy1 =	0.00227;
p_Hy2 =	-0.00772;
p_Hy3 =	-0.12814;
p_Vy1 =	0.14237;
p_Vy2 =	-0.17287;
p_Vy3 =	-1.49583;
p_Vy4 =	4.55061;

% [LONGITUDINAL COEFFICIENTS]
p_Cx1 = 1.43990;
p_Dx1 =	2.59060;
p_Dx2 =	-0.36627;
p_Ex1 =	-0.24355;
p_Ex2 =	-0.66953;
p_Ex3 =	-3.71110;
p_Ex4 =	0.37836;
p_Kx1 =	36.76960;
p_Kx2 =	-23.37320;
p_Kx3 =	-0.45230;
p_Hx1 =	0.00098;
p_Hx2 =	0.00014;
p_Vx1 =	-0.04913;
p_Vx2 =	0.02482;

== matlab function EVX_Car_Model/EVX Vehicle Model/Subsystem1/MATLAB Function8 ==
  data: Fz input; Fxo output; kappa input; alpha input; gam input; Fzo input; Ro input; Fyo output; Mzo output; q_Bz1 input; q_Bz2 input; q_Bz3 input; q_Bz4 input; q_Bz5 input; q_Bz9 input; q_Bz10 input; q_Cz1 input; q_Dz1 input; q_Dz2 input; q_Dz3 input; q_Dz4 input; q_Dz6 input; q_Dz7 input; q_Dz8 input; q_Dz9 input; q_Ez1 input; q_Ez2 input; q_Ez3 input; q_Ez4 input; q_Ez5 input; q_Hz1 input; q_Hz2 input; q_Hz3 input; q_Hz4 input; p_Cy1 input; p_Dy1 input; p_Dy2 input; p_Dy3 input; p_Ey1 input; p_Ey2 input; p_Ey3 input; p_Ey4 input; p_Ky1 input; p_Ky2 input; p_Ky3 input; p_Hy1 input; p_Hy2 input; p_Hy3 input; p_Vy1 input; p_Vy2 input; p_Vy3 input; p_Vy4 input; p_Cx1 input; p_Dx1 input; p_Dx2 input; p_Ex1 input; p_Ex2 input; p_Ex3 input; p_Ex4 input; p_Kx1 input; p_Kx2 input; p_Kx3 input; p_Hx1 input; p_Hx2 input; p_Vx1 input; p_Vx2 input; car_mu_scaling input; run_info input
function [Fxo,Fyo,Mzo] = Pacejka_Tyre_Model(Fz,kappa,alpha,gam,Fzo,Ro,...
    q_Bz1,q_Bz2,q_Bz3,q_Bz4,q_Bz5,q_Bz9,q_Bz10,q_Cz1,q_Dz1,...
    q_Dz2,q_Dz3,q_Dz4,q_Dz6,q_Dz7,q_Dz8,q_Dz9,q_Ez1,q_Ez2,q_Ez3,q_Ez4,q_Ez5,...
    q_Hz1,q_Hz2,q_Hz3,q_Hz4,p_Cy1,p_Dy1,p_Dy2,p_Dy3,p_Ey1,p_Ey2,p_Ey3,...
    p_Ey4,p_Ky1,p_Ky2,p_Ky3,p_Hy1,p_Hy2,p_Hy3,p_Vy1,p_Vy2,p_Vy3,p_Vy4,...
    p_Cx1,p_Dx1,p_Dx2,p_Ex1,p_Ex2,p_Ex3,p_Ex4,p_Kx1,p_Kx2,p_Kx3,p_Hx1,...
    p_Hx2,p_Vx1,p_Vx2,car_mu_scaling,run_info)
% Pacejka '96 tyre model
%
% Inputs:
% Fz:       normal force (N)
% kappa:    slip ratio (% between -1 and 1) +ve is driving, -ve is braking
% alpha:    slip angle (rad) +ve alpha generates +ve Fyo
% gam:      inclanation angle/camber (rad) +ve indicates top of tyre tipped
%           right
% Outputs:
% Fxo:      Longitudinal force (N)
% Fyo:      Lateral force (N)
% Mzo:      Aligning moment (Nm)


%% tyre coefficients
% each different type of tyre holds different scaling coefficients, load 
% these here Also loaded are unloaded tyre radius and nominal wheel load

% unpack the structure holding the coefficients
% Get the field names of the structure
% fields = fieldnames(carpacejka_coefs, '-full');

% for ii = 1:length(fields)
%     thisField = fields{ii};
%     create_variable = sprintf('%s = carpacejka_coefs%s;', thisField, thisField);
%     eval(create_variable);
% end
% clear('ii', 'thisField');
% clear('fields', 'create_variable');

%% register track conditions
% scaling factors affected by wet/dry conditions

    lambda_mux = 1; % peak friction coefficient
    lambda_muy = 1; % peak friction coefficient

% modify with user scaling factor
lambda_mux = lambda_mux*car_mu_scaling;
lambda_muy = lambda_muy*car_mu_scaling;

%% scaling factors
% default values for these values is 1 (except lambda_muV=0)
lambda_Fzo = 1; % nominal rated load
lambda_muV = 0; % with slip speed Vx decaying friction
lambda_Kx = 1; % brake slip stiffness
lambda_Ky = 1; % cornering stiffness
lambda_Cx = 1; % shape factor
lambda_Cy = 1; % shape factor
lambda_Ex = 1; % curvature factor
lambda_Ey = 1; % curvature factor
lambda_Hx = 1; % horizontal shift
lambda_Hy = 1; % horizontal shift
lambda_Vx = 1; % vertical shift
lambda_Vy = 1; % vertical shift
lambda_Kygam = 1; % camber force stiffness
lambda_Kzgam = 1; % camber torque stiffness
lambda_t = 1; % pneumatic trail
lambda_Mr = 1; % residual torque
lambda_ygam = 1;

if ~isrow(kappa) || ~isrow(alpha) || ~isrow(gam)
    kappa = transpose(kappa);
    alpha = transpose(alpha);
    gam = transpose(gam);
end

for ii=1:length(Fz)
    %% derived inputs
    dfz = (Fz(ii)-Fzo)/Fzo; % normalised change in vertical load
    
    %% longitudinal force (pure longitudinal slip)
    S_Vx = Fz(ii)*(p_Vx1+p_Vx2*dfz)*lambda_Vx*lambda_mux;
    S_Hx = (p_Hx1+p_Hx2*dfz)*lambda_Hx;
    kappa_x = kappa + S_Hx;
    K_xk = Fz(ii)*(p_Kx1+p_Kx2*dfz)*exp(-p_Kx3*dfz)*lambda_Kx;
    E_x = (p_Ex1+p_Ex2*dfz+p_Ex3*dfz^2)*(1-p_Ex4*sign(kappa_x))*lambda_Ex;
    mu_x = (p_Dx1+p_Dx2*dfz)*lambda_mux;
    D_x = mu_x*Fz(ii);
    C_x = p_Cx1*lambda_Cx;
    B_x = K_xk/(C_x*D_x);
    Fxo = D_x*sin(C_x*atan(B_x*kappa_x - E_x*(B_x*kappa_x-atan(B_x*kappa_x)))) + S_Vx;
    
    %% lateral force (pure lateral slip)
    gam_y = gam*lambda_ygam;
    C_y = p_Cy1*lambda_Cy;
    mu_y = (p_Dy1+p_Dy2*dfz)*(1-p_Dy3*gam^2)*lambda_muy;
    D_y = mu_y*Fz(ii);
    S_Hy = (p_Hy1+p_Hy2*dfz+p_Hy3*gam)*lambda_Hy;
    alpha_y = alpha + S_Hy;
    E_y = (p_Ey1+p_Ey2*dfz)*(1-(p_Ey3+p_Ey4*gam_y)*sign(alpha_y))*lambda_Ey;
    K_ya = p_Ky1*Fzo*sin(2*atan(Fz(ii)/(p_Ky2*Fzo*lambda_Fzo)))*(1-p_Ky3*abs(gam))*lambda_Fzo*lambda_Ky;
    B_y = K_ya/(C_y*D_y);
    S_Vy = Fz(ii)*((p_Vy1+p_Vy2*dfz)+(p_Vy3+p_Vy4*dfz)*gam*lambda_Vy*lambda_Kygam);
    Fyo = D_y*sin(C_y*atan(B_y*alpha_y - E_y*(B_y*alpha_y-atan(B_y*alpha_y)))) + S_Vy;
    
    %% aligning torque (pure side slip)
    B_t = (q_Bz1+q_Bz2*dfz+q_Bz3*dfz^2)*(1+q_Bz4*gam*q_Bz5*abs(gam))*lambda_Ky/lambda_muy;
    C_t = q_Cz1;
    D_t = (q_Dz1+q_Dz2*dfz)*(1+q_Dz3*gam+q_Dz4*gam^2)*Ro*lambda_t/Fzo;
    S_Ht = q_Hz1+q_Hz2*dfz+(q_Hz3+q_Hz4*dfz)*gam;
    alpha_t = alpha + S_Ht;
    E_t = (q_Ez1+q_Ez2*dfz+q_Ez3*dfz^2)*(1+(q_Ez4+q_Ez5*gam)*atan(B_t*C_t*alpha_t));
    B_r = (q_Bz9*lambda_Ky/lambda_muy+q_Bz10*B_y*C_y);
    D_r = Fz(ii)*((q_Dz6+q_Dz7*dfz)+(q_Dz8+q_Dz9*dfz)*gam)*Ro*lambda_muy*lambda_Mr;
    S_Hf = S_Hy + S_Vy/K_ya;
    alpha_r = alpha + S_Hf;
    Mzr = D_r*cos(atan(B_r*alpha_r))*cos(alpha);
    t = D_t*cos(C_t*atan(B_t*alpha_t-E_t*(B_t*alpha_t-atan(B_t*alpha_t))))*cos(alpha);
    Mzo = -t*Fyo + Mzr;
    
end

== matlab function EVX_Car_Model/EVX Vehicle Model/Subsystem1/MATLAB Function ==
  data: x input; F_z output; xdot input; k input; c input
function F_z = fcn(x,xdot,k,c)

F_z = k * x + c * xdot;

== matlab function EVX_Car_Model/EVX Vehicle Model/Car_Parameters/MATLAB Function21 ==
  data: whatever input; k_SFR output; Owen input; wants input; k_SFL output; k_SRR output; k_SRL output; c_SFR output; c_SFL output; c_SRR output; c_SRL output; k_TFR output; k_TFL output; k_TRR output; k_TRL output; c_TFR output; c_TFL output; c_TRR output; c_TRL output; k_RF output; k_RR output; k_FRIC output; c_RF output; c_RR output; c_FRIC output; gamma_FR output; gamma_FL output; gamma_RR output; gamma_RL output; I_WFR output; I_WFL output; I_WRR output; I_WRL output
function [k_SFR,k_SFL,k_SRR,k_SRL,c_SFR,c_SFL,c_SRR,c_SRL,k_TFR,k_TFL,...
    k_TRR,k_TRL,c_TFR,c_TFL,c_TRR,c_TRL,k_RF,k_RR,k_FRIC,c_RF,c_RR,...
    c_FRIC,gamma_FR,gamma_FL,gamma_RR,gamma_RL,I_WFR,I_WFL,I_WRR,I_WRL]...
    = Suspension_Mapping(whatever,Owen,wants)

% Suspension Stifnesses
k_SFR = 2000; %suspension stiffness front right (N/m)
k_SFL = 2000; %suspension stiffness front left (N/m)
k_SRR = 2000; %suspension stiffness rear right (N/m)
k_SRL = 2000; %suspension stiffness rear left (N/m)

% Tire Stifnesses
k_TFR = 15000; %tire stiffness front right (N/m)
k_TFL = 15000; %tire stiffness front left (N/m)
k_TRR = 15000; %tire stiffness rear right (N/m)
k_TRL = 15000; %tire stiffness rear left (N/m)

% Suspension Damping Coefficients
c_SFR = 1000; %suspension damping coefficient front right (Ns/m)
c_SFL = 1000; %suspension damping coefficient front left (Ns/m)
c_SRR = 1000; %suspension damping coefficientv rear right (Ns/m)
c_SRL = 1000; %suspension damping coefficient rear left (Ns/m)

% Tire Damping Coefficients
c_TFR = 500; %tire damping coefficient front right (Ns/m)
c_TFL = 500; %tire damping coefficient front left (Ns/m)
c_TRR = 500; %tire damping coefficientv rear right (Ns/m)
c_TRL = 500; %tire damping coefficient rear left (Ns/m)

% Roll Bar Stiffnesses
k_RF = 0; %front
k_RR = 0; %rear
k_FRIC = 0; %front to rear

% Roll Bar Damping
c_RF = 0; %front
c_RR = 0; %rear
c_FRIC = 0; %front to rear

% Camber (deg) (tilt right positive)
gamma_FRd = 0;
gamma_FLd = 0;
gamma_RRd = 0;
gamma_RLd = 0;

% Camber (Rad)
Deg2Rad = 0.0174533;
gamma_FR = gamma_FRd * Deg2Rad;
gamma_FL = gamma_FLd * Deg2Rad;
gamma_RR = gamma_RRd * Deg2Rad;
gamma_RL = gamma_RLd * Deg2Rad;

% Wheel Inertias
I_WFR = 10;
I_WFL = 10;
I_WRR = 10;
I_WRL = 10;

== matlab function EVX_Car_Model/EVX Vehicle Model/MATLAB Function22 ==
  data: g output
function g  = Environment_Parameters

g = 9.81;

== matlab function EVX_Car_Model/EVX Vehicle Model/Chassis Vertical Dynamics/MATLAB Function22 ==
  data: g input; F_zWFR output; m_WFR input; m_WFL input; m_WRR input; m_WRL input; F_zWFL output; F_zWRR output; F_zWRL output
function [F_zWFR,F_zWFL,F_zWRR,F_zWRL] = fcn(g,m_WFR,m_WFL,m_WRR,m_WRL)

F_zWFR = -g * m_WFR;
F_zWFL = -g * m_WFL;
F_zWRR = -g * m_WRR;
F_zWRL = -g * m_WRL;

== matlab function EVX_Car_Model/EVX Vehicle Model/MATLAB Function23 ==
  data: v_y input; ratio_FR output; angle_FR output; ratio_FL output; angle_FL output; ratio_RR output; angle_RR output; ratio_RL output; angle_RL output; v_x input; a input; b input; d_F input; e_F input; d_R input; e_R input; Idot_z input; r_FR input; r_FL input; r_RR input; r_RL input; S_FR input; S_FL input; S_RR input; S_RL input; w_FR input; w_FL input; w_RR input; w_RL input
function [ratio_FR,angle_FR,ratio_FL,angle_FL,ratio_RR,angle_RR,ratio_RL,...
    angle_RL] = Tyre_Slips(v_y,v_x,a,b,d_F,e_F,d_R,e_R,Idot_z,r_FR,r_FL,...
    r_RR,r_RL,S_FR,S_FL,S_RR,S_RL,w_FR,w_FL,w_RR,w_RL)

beta = atan(v_y/v_x);

v_yFR = v_y + Idot_z * a;
v_yFL = v_y + Idot_z * a;
v_yRR = v_y + Idot_z * -b;
v_yRL = v_y + Idot_z * -b;

v_xFR = v_x - Idot_z * e_F;
v_xFL = v_x - Idot_z * -d_F;
v_xRR = v_x - Idot_z * e_R;
v_xRL = v_x - Idot_z * -d_R;

beta_FR = atan(v_yFR/v_xFR);
beta_FL = atan(v_yFL/v_xFL);
beta_RR = atan(v_yRR/v_xRR);
beta_RL = atan(v_yRL/v_xRL);

w0_FR = v_x / r_FR;
w0_FL = v_x / r_FL;
w0_RR = v_x / r_RR;
w0_RL = v_x / r_RL;

ratio_FR = (w_FR - w0_FR)/w0_FR;
angle_FR = beta_FR - S_FR;
ratio_FL = (w_FL - w0_FL)/w0_FL;
angle_FL = beta_FL - S_FL;
ratio_RR = (w_RR - w0_RR)/w0_RR;
angle_RR = beta_RR - S_RR;
ratio_RL = (w_RL - w0_RL)/w0_RL;
angle_RL = beta_RL - S_RL;

% ratio_FR = 0;
% angle_FR = 0;
% ratio_FL = 0;
% angle_FL = 0;
% ratio_RR = 0;
% angle_RR = 0;
% ratio_RL = 0;
% angle_RL = 0;

== matlab function EVX_Car_Model/EVX Vehicle Model/MATLAB Function25 ==
  data: r output; F_x input; T input; I input; wdot output; r_static input; w input
function [r,wdot] = Wheel_Dynamics(F_x,T,I,r_static,w)

r = r_static + 0.005 .* w;

wdot = (T - F_x .* r)./I;
